simulink model "TwoCellImplementation"  (R2021b)
settings: Solver=VariableStepAuto  StartTime=0.0  StopTime=1000  RelTol=1e-3
libraries: spsVoltageMeasurementLib x6, spsDiodeLib x2, spsSeriesRLCBranchLib x2, spsGroundLib x1, spsLinearTransformerLib x1, spsMosfetLib x1, spspowerguiLib x1
settings Model: Creator=HP  LastModifiedBy=rajra
settings SolverCC: AlgebraicLoopSolver=TrustRegion
settings DebuggingCC: SFMachineParentedDataDiag=warning

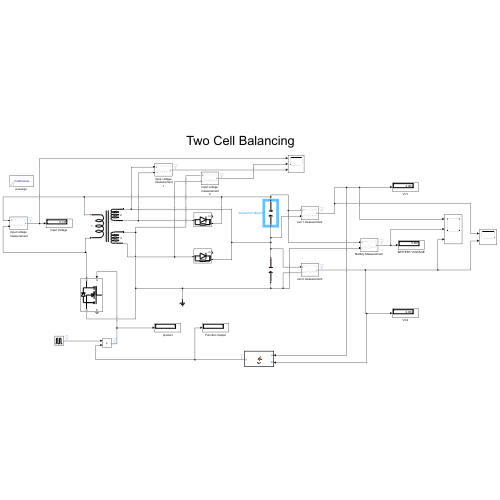
[thumbnail: Simulink's stored preview of the top-level diagram]
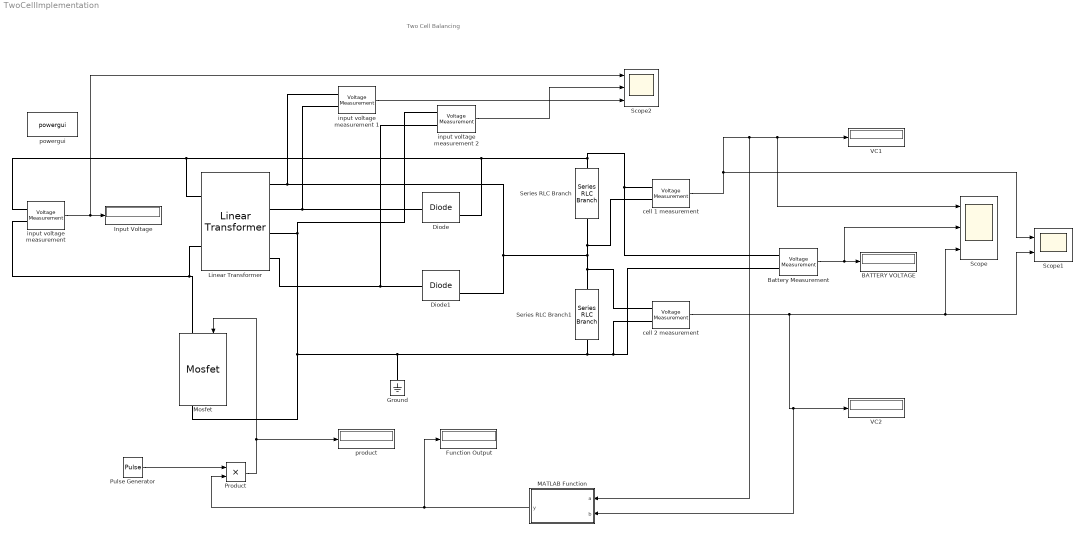
== system TwoCellImplementation ==
  note: Two Cell Balancing
  BATTERY VOLTAGE : Display
  "Battery Measurement " : spsVoltageMeasurementLib/Voltage Measurement  PhasorSimulation=off  OutputType=Complex  PSBequivalent=0
  Diode : spsDiodeLib/Diode  Ron=0.001  Lon=0  Vf=0.8  IC=0  UseSnubber=0  Rs=500  Cs=250e-9  Measurements=on
  Diode1 : spsDiodeLib/Diode  Ron=0.001  Lon=0  Vf=0.8  IC=0  UseSnubber=0  Rs=500  Cs=250e-9  Measurements=on
  Function Output : Display
  Ground : spsGroundLib/Ground  LConnTagsString=a
  Input Voltage : Display
  Linear Transformer : spsLinearTransformerLib/Linear Transformer  UNITS=SI  NominalPower=[100 55000]  winding1=[10 0.02 45e-6]  winding2=[5 0.02 288e-6]  ThreeWindings=on  winding3=[5 0.02 288e-6]  RmLm=[1.0805e+06 2866]  Measurements=None  DataType=on
  MATLAB Function : MATLAB Function  TreatAsAtomicUnit=on
  Mosfet : spsMosfetLib/Mosfet  Ron=1.5  Lon=0  Rd=2  Vfd=0  IC=0  Rs=1500  Cs=288e-7  Measurements=on
  Product : Product
  Pulse Generator : DiscretePulseGenerator  PulseType=Time based  Period=10  PulseWidth=50
  Scope : Scope  NumInputPorts=3
  Scope1 : Scope  NumInputPorts=2
  Scope2 : Scope  NumInputPorts=3
  Series RLC Branch : spsSeriesRLCBranchLib/Series RLC Branch  LConnTagsString=__new0  RConnTagsString=__new0  BranchType=C  Resistance=1  Inductance=1e-3  SetiL0=off  InitialCurrent=0  Capacitance=5  Setx0=on  InitialVoltage=2.6  Measurements=None
  Series RLC Branch1 : spsSeriesRLCBranchLib/Series RLC Branch  LConnTagsString=__new0  RConnTagsString=__new0  BranchType=C  Resistance=1  Inductance=1e-3  SetiL0=off  InitialCurrent=0  Capacitance=5  Setx0=on  InitialVoltage=3.4  Measurements=Branch voltage
  "VC1 " : Display
  VC2 : Display
  "cell 1 measurement " : spsVoltageMeasurementLib/Voltage Measurement  PhasorSimulation=off  OutputType=Complex  PSBequivalent=0
  "cell 2 measurement " : spsVoltageMeasurementLib/Voltage Measurement  PhasorSimulation=off  OutputType=Complex  PSBequivalent=0
  "input voltage measurement " : spsVoltageMeasurementLib/Voltage Measurement  PhasorSimulation=off  OutputType=Complex  PSBequivalent=0
  input voltage measurement 1 : spsVoltageMeasurementLib/Voltage Measurement  PhasorSimulation=off  OutputType=Complex  PSBequivalent=0
  input voltage measurement 2 : spsVoltageMeasurementLib/Voltage Measurement  PhasorSimulation=off  OutputType=Complex  PSBequivalent=0
  powergui : spspowerguiLib/powergui  Priority=1  SimulationMode=Continuous  SampleTime=50e-6  frequency=60  Iterations=50  frequencyindice=0  Pbase=100e6  ErrMax=1e-4  UnitsV=kV  UnitsW=MW  buscounter=0  FunctionMessages=off  echomessages=off  EnableUseOfTLC=off  CurrentSourceSwitches=off  DisableSnubberDevices=off  DisableRonSwitches=off  DisableVfSwitches=off  DisplayEquations=off  AutomaticDiscreteSolvers=off  SolverType=Tustin/Backward Euler (TBE)  Interpol=off  ExternalGateDelay=off  methode=off  Ts=100  x0status=blocks  SPID=on  SwTol=0  HookPort=off  NonlinearTolerance=1e-4  nMaxIteration=100  ContinueOnMaxIteration=off  RestoreLinks=warning  ResistiveCurrentMeasurement=off  Frange=[0:2:500]  Ylog=off  Xlog=on  ShowGrid=off  save=off  variable=ZData  structure=0  ZoomFFT=off  StartTime=0.0  cycles=1  DisplayStyle=1  fundamental=60  FreqAxis=off  MaxFrequency=1000  frequencyindicesteady=1  RmsSteady=1  display=off
  "product " : Display
  wires:
  Pulse Generator/1 -> Product/1
  Product/1 -> "product "/1, Mosfet/1
  MATLAB Function/1(y) -> Product/2, Function Output/1
  "cell 1 measurement "/1 -> MATLAB Function/1(a), Scope/1, "VC1 "/1, Scope1/1
  "cell 2 measurement "/1 -> Scope1/2, Scope/3, MATLAB Function/2(b), VC2/1
  "Battery Measurement "/1 -> Scope/2, BATTERY VOLTAGE/1
  "input voltage measurement "/1 -> Scope2/1, Input Voltage/1
  input voltage measurement 1/1 -> Scope2/3
  input voltage measurement 2/1 -> Scope2/2
  connections:
  Linear Transformer/RConn2 -- input voltage measurement 1/LConn2 -- Diode/LConn1
  Linear Transformer/RConn4 -- input voltage measurement 2/LConn2 -- Diode1/LConn1
  Diode/RConn1 -- Linear Transformer/LConn1 -- "input voltage measurement "/LConn1 -- "Battery Measurement "/LConn1 -- "cell 1 measurement "/LConn1 -- Series RLC Branch/LConn1
  input voltage measurement 1/LConn1 -- Linear Transformer/RConn1 -- Diode1/RConn1 -- Series RLC Branch/RConn1 -- "cell 1 measurement "/LConn2 -- Series RLC Branch1/LConn1 -- "cell 2 measurement "/LConn1
  Linear Transformer/LConn2 -- "input voltage measurement "/LConn2 -- Mosfet/LConn1
  Linear Transformer/RConn3 -- Ground/LConn1 -- "Battery Measurement "/LConn2 -- "cell 2 measurement "/LConn2 -- Series RLC Branch1/RConn1 -- Mosfet/RConn1 -- input voltage measurement 2/LConn1

== matlab function TwoCellImplementation/MATLAB Function ==
  data: a input; y output; b input
function y = fcn(a,b)
if(a==b)
    y = 0;
else
    y = 1;
end
